simulink model "Simulador_PID"  (R2023b)
settings: Solver=VariableStepAuto  StartTime=0.0  StopTime=10  RelTol=1e-3
InitFcn:
  | Parametros;
undefined symbols (not defined in the file): Jt, Mt
settings Model: Creator=iangr  LastModifiedBy=iangr

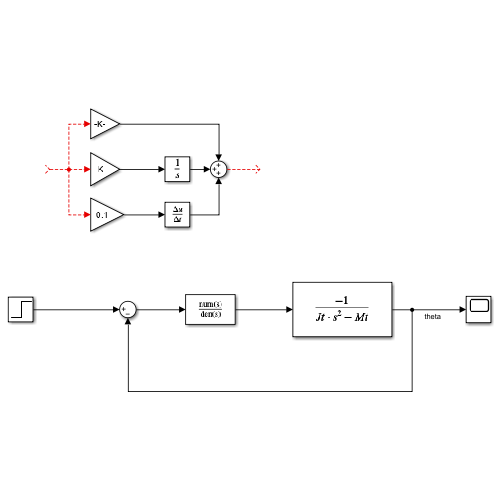
[thumbnail: Simulink's stored preview of the top-level diagram]
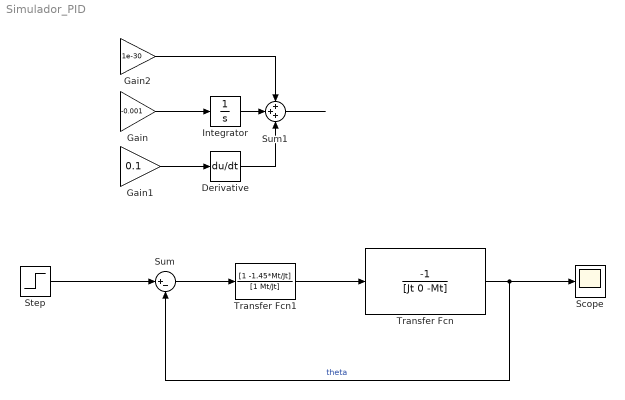
== system Simulador_PID ==
  Derivative : Derivative
  Gain : Gain  Gain=-0.001
  Gain1 : Gain  Gain=0.1
  Gain2 : Gain  Gain=1e-30
  Integrator : Integrator
  Scope : Scope
  Step : Step  SampleTime=0
  Sum : Sum  Inputs=|+-
  Sum1 : Sum  Inputs=+++
  Transfer Fcn : TransferFcn  Numerator=[-1]  Denominator=[Jt 0 -Mt]
  Transfer Fcn1 : TransferFcn  Numerator=[1 -1.45*Mt/Jt]  Denominator=[1 Mt/Jt]
  wires:
  Transfer Fcn/1 -> Scope/1, Sum/2  "theta"
  Step/1 -> Sum/1
  Gain/1 -> Integrator/1
  Integrator/1 -> Sum1/2
  ? -> Gain1/1, Gain/1, Gain2/1
  Sum1/1 -> ?
  Gain1/1 -> Derivative/1
  Gain2/1 -> Sum1/1
  Derivative/1 -> Sum1/3
  Sum/1 -> Transfer Fcn1/1
  Transfer Fcn1/1 -> Transfer Fcn/1
